simulink model "tadpole_dynamic_open_loop1"  (R2019b)
settings: Solver=ode4  StartTime=0.0  StopTime=sim_time  FixedStep=0.001  RelTol=1e-2
values from neighbouring files (symbols this model uses):
  C_alpha = 1000*ones(runcycle,1)    [rand_par.m]    (also in whole_par.m = 1000; whole_par_bias.m = 1000)
  C_beta = 50*ones(runcycle,1)    [rand_par.m]    (also in whole_par.m = 50; whole_par_bias.m = 50)
  Cd = 0.25*ones(runcycle,1)    [rand_par.m]    (also in whole_par.m = 0.25; whole_par_bias.m = 0.25)
  delta_fL = -1*ones(runcycle,1)    [rand_par.m]    (also in whole_par.m = -1; whole_par_bias.m = -1)
  delta_fR = 3.5*ones(runcycle,1)    [rand_par.m]    (also in whole_par.m = 3.5; whole_par_bias.m = 3.5)
  FA = 1*ones(runcycle,1)    [rand_par.m]    (also in whole_par.m = 1; whole_par_bias.m = 1)
  h = [ h(1:j-1) ; h(j+1:m)]    [UMDIRECT.m]    (also in whole_par.m = 0.4896; whole_par_bias.m = 0.4896)
  I_f_wheel = 0.3    [whole_par.m]    (also in whole_par_bias.m)
  I_r_wheel = 0.5    [whole_par.m]    (also in whole_par_bias.m)
  I_x = 12.1*ones(runcycle,1)    [rand_par.m]    (also in whole_par.m = 12.1; whole_par_bias.m = 12.1)
  I_y = 36.7*ones(runcycle,1)    [rand_par.m]    (also in whole_par.m = 36.7; whole_par_bias.m = 36.7)
  I_z = 50*DOE(:,2)    [rand_par.m]    (also in whole_par.m = 50; whole_par_bias.m = 60)
  k_z = 30000*ones(runcycle,1)    [rand_par.m]    (also in whole_par.m = 30000; whole_par_bias.m = 30000)
  l_1 = 0.724    [whole_par.m]    (also in whole_par_bias.m)
  l_2 = 0.719    [whole_par.m]    (also in whole_par_bias.m)
  m = m - 1    [UMDIRECT.m]    (also in rand_par.m = 48.3*DOE(:,1); whole_par.m = 48.3; whole_par_bias.m = 60)
  mu_dp = 0.8*ones(runcycle,1)    [rand_par.m]    (also in whole_par.m = 0.8; whole_par_bias.m = 0.8)
  mu_lp = 0.8*ones(runcycle,1)    [rand_par.m]    (also in whole_par.m = 0.8; whole_par_bias.m = 0.8)
  mu_rolling_1 = 0.009*ones(runcycle,1)    [rand_par.m]    (also in whole_par.m = 0.009; whole_par_bias.m = 0.009)
  mu_rolling_2 = 0.0005*ones(runcycle,1)    [rand_par.m]    (also in whole_par.m = 0.0005; whole_par_bias.m = 0.0005)
  R_0 = 0.335*ones(runcycle,1)    [rand_par.m]    (also in whole_par.m = 0.335; whole_par_bias.m = 0.335)
  rho = 1.225*ones(runcycle,1)    [rand_par.m]    (also in whole_par.m = 1.225; whole_par_bias.m = 1.225)
  SAP = 0.01*ones(runcycle,1)    [rand_par.m]    (also in whole_par.m = 0.01; whole_par_bias.m = 0.01)
  V_wind = 0*ones(runcycle,1)    [rand_par.m]    (also in whole_par.m = 0; whole_par_bias.m = 0)
libraries: simulink_extras x10, simulink x4
(part 3 of 4)

== system tadpole_dynamic_open_loop1/Vehicle Model/resistance calculation/Rear Traction add up/Fm<0/Switch Case Action Subsystem15 ==
  "value " : Inport
  Action Port : ActionPort  ActionPortLabel=case [ 1 ]:
  Merge1 : Merge  Inputs=3
  Switch Case Action Subsystem6 : Subsystem  TreatAsAtomicUnit=on
  Switch Case Action Subsystem7 : Subsystem  TreatAsAtomicUnit=on
  Switch Case Action Subsystem8 : Subsystem  TreatAsAtomicUnit=on
  Switch Case3 : SwitchCase  CaseConditions={1,-1}
  Out1 : Outport  VectorParamsAs1DForOutWhenUnconnected=off
  wires:
  Switch Case Action Subsystem7/1(Out1) -> Merge1/2
  Switch Case Action Subsystem6/1(Out1) -> Merge1/1
  [minus] -> Switch Case Action Subsystem7/1("value ")
  Switch Case Action Subsystem8/1(Out1) -> Merge1/3
  Switch Case3/2 -> Switch Case Action Subsystem7/Action  "m<b"
  [add] -> Switch Case Action Subsystem6/1("value ")
  Switch Case3/3 -> Switch Case Action Subsystem8/Action  "m=b"
  [minus] -> Switch Case Action Subsystem8/1("value ")
  Switch Case3/1 -> Switch Case Action Subsystem6/Action  "m>b"
  Merge1/1 -> Out1/1
  "value "/1 -> Switch Case3/1

== system tadpole_dynamic_open_loop1/Vehicle Model/resistance calculation/Rear Traction add up/Fm<0/Switch Case Action Subsystem6 ==
  "value " : Inport
  Action Port : ActionPort  ActionPortLabel=case [ -1 ]:
  Constant1 : Constant  Value=0
  Merge2 : Merge  Inputs=3
  Switch Case Action Subsystem10 : Subsystem  TreatAsAtomicUnit=on
  Switch Case Action Subsystem11 : Subsystem  TreatAsAtomicUnit=on
  Switch Case Action Subsystem9 : Subsystem  TreatAsAtomicUnit=on
  Switch Case4 : SwitchCase  CaseConditions={1,-1}
  Out1 : Outport  VectorParamsAs1DForOutWhenUnconnected=off
  wires:
  "value "/1 -> Switch Case4/1
  Switch Case4/2 -> Switch Case Action Subsystem10/Action  "m<b"
  [minus] -> Switch Case Action Subsystem10/1("value ")
  Switch Case Action Subsystem10/1(Out1) -> Merge2/2
  [add] -> Switch Case Action Subsystem9/1("value ")
  Switch Case4/1 -> Switch Case Action Subsystem9/Action  "m>b"
  Switch Case Action Subsystem9/1(Out1) -> Merge2/1
  Switch Case4/3 -> Switch Case Action Subsystem11/Action  "m=b"
  Constant1/1 -> Switch Case Action Subsystem11/1("value ")
  Switch Case Action Subsystem11/1(Out1) -> Merge2/3
  Merge2/1 -> Out1/1

== system tadpole_dynamic_open_loop1/Vehicle Model/resistance calculation/Rear Traction add up/Fm<0/Switch Case Action Subsystem7 ==
  "value " : Inport
  Action Port : ActionPort  ActionPortLabel=default:
  Constant1 : Constant  Value=0
  Constant2 : Constant  Value=0
  Merge3 : Merge  Inputs=3
  Switch Case Action Subsystem12 : Subsystem  TreatAsAtomicUnit=on
  Switch Case Action Subsystem13 : Subsystem  TreatAsAtomicUnit=on
  Switch Case Action Subsystem14 : Subsystem  TreatAsAtomicUnit=on
  Switch Case5 : SwitchCase  CaseConditions={1,-1}
  Out1 : Outport  VectorParamsAs1DForOutWhenUnconnected=off
  wires:
  "value "/1 -> Switch Case5/1
  Switch Case5/1 -> Switch Case Action Subsystem14/Action  "m>b"
  Switch Case Action Subsystem14/1(Out1) -> Merge3/1
  Switch Case Action Subsystem12/1(Out1) -> Merge3/2
  Constant1/1 -> Switch Case Action Subsystem12/1("value ")
  Switch Case Action Subsystem13/1(Out1) -> Merge3/3
  Switch Case5/3 -> Switch Case Action Subsystem13/Action  "m=b"
  Switch Case5/2 -> Switch Case Action Subsystem12/Action  "m<b"
  [add] -> Switch Case Action Subsystem14/1("value ")
  Constant2/1 -> Switch Case Action Subsystem13/1("value ")
  Merge3/1 -> Out1/1

== system tadpole_dynamic_open_loop1/Vehicle Model/resistance calculation/Rear Traction add up/Fm>=0/Switch Case Action Subsystem6 ==
  "value " : Inport
  In2 : Inport  Port=2
  In3 : Inport  Port=3
  Action Port : ActionPort  ActionPortLabel=case [ -1 ]:
  Constant : Constant  Value=2
  Constant1 : Constant  Value=0
  Merge2 : Merge  Inputs=3
  Switch Case Action Subsystem10 : Subsystem  TreatAsAtomicUnit=on
  Switch Case Action Subsystem11 : Subsystem  TreatAsAtomicUnit=on
  Switch Case Action Subsystem9 : Subsystem  TreatAsAtomicUnit=on
  Switch Case4 : SwitchCase  CaseConditions={1,-1}
  Out1 : Outport  VectorParamsAs1DForOutWhenUnconnected=off
  Out2 : Outport  Port=2  VectorParamsAs1DForOutWhenUnconnected=off
  wires:
  "value "/1 -> Switch Case4/1
  Switch Case4/2 -> Switch Case Action Subsystem10/Action  "V-"
  [minus_2] -> Switch Case Action Subsystem10/1("value ")
  Switch Case Action Subsystem10/1(Out1) -> Merge2/2
  [minus_2] -> Switch Case Action Subsystem9/1("value ")
  Switch Case4/1 -> Switch Case Action Subsystem9/Action  "V+"
  Switch Case Action Subsystem9/1(Out1) -> Merge2/1
  Switch Case4/3 -> Switch Case Action Subsystem11/Action  "V=0"
  Constant1/1 -> Switch Case Action Subsystem11/1("value ")
  Switch Case Action Subsystem11/1(Out1) -> Merge2/3
  Merge2/1 -> Out1/1
  In2/1 -> [add_2]
  In3/1 -> [minus_2]
  Constant/1 -> Out2/1

== system tadpole_dynamic_open_loop1/Vehicle Model/resistance calculation/Rear Traction add up/Fm>=0/Switch Case Action Subsystem7 ==
  "value " : Inport
  In2 : Inport  Port=2
  In3 : Inport  Port=3
  Action Port : ActionPort  ActionPortLabel=default:
  Constant : Constant  Value=3
  Constant2 : Constant  Value=0
  Merge3 : Merge  Inputs=3
  Switch Case Action Subsystem12 : Subsystem  TreatAsAtomicUnit=on
  Switch Case Action Subsystem13 : Subsystem  TreatAsAtomicUnit=on
  Switch Case Action Subsystem14 : Subsystem  TreatAsAtomicUnit=on
  Switch Case5 : SwitchCase  CaseConditions={1,-1}
  Out1 : Outport  VectorParamsAs1DForOutWhenUnconnected=off
  Out2 : Outport  Port=2  VectorParamsAs1DForOutWhenUnconnected=off
  wires:
  "value "/1 -> Switch Case5/1
  Switch Case5/1 -> Switch Case Action Subsystem14/Action  "m>b"
  Switch Case Action Subsystem14/1(Out1) -> Merge3/1
  Switch Case Action Subsystem12/1(Out1) -> Merge3/2
  [minus_3] -> Switch Case Action Subsystem12/1("value ")
  Switch Case Action Subsystem13/1(Out1) -> Merge3/3
  Switch Case5/3 -> Switch Case Action Subsystem13/Action  "m=b"
  Switch Case5/2 -> Switch Case Action Subsystem12/Action  "m<b"
  [minus_3] -> Switch Case Action Subsystem14/1("value ")
  Constant2/1 -> Switch Case Action Subsystem13/1("value ")
  Merge3/1 -> Out1/1
  In2/1 -> [add_3]
  In3/1 -> [minus_3]
  Constant/1 -> Out2/1

== system tadpole_dynamic_open_loop1/Vehicle Model/resistance calculation/Rear Traction add up/Fm>=0/m>b ==
  "velocity sign " : Inport
  add : Inport  Port=2
  "minus " : Inport  Port=3
  Action Port : ActionPort  ActionPortLabel=case [ 1 ]:
  Constant : Constant
  Merge1 : Merge  Inputs=3
  Switch Case Action Subsystem6 : Subsystem  TreatAsAtomicUnit=on
  Switch Case Action Subsystem7 : Subsystem  TreatAsAtomicUnit=on
  Switch Case Action Subsystem8 : Subsystem  TreatAsAtomicUnit=on
  Switch Case3 : SwitchCase  CaseConditions={1,-1}
  Out1 : Outport  VectorParamsAs1DForOutWhenUnconnected=off
  Out2 : Outport  Port=2  VectorParamsAs1DForOutWhenUnconnected=off
  wires:
  Switch Case Action Subsystem7/1(Out1) -> Merge1/2
  Switch Case Action Subsystem6/1(Out1) -> Merge1/1
  [add_1] -> Switch Case Action Subsystem7/1("value ")
  Switch Case Action Subsystem8/1(Out1) -> Merge1/3
  Switch Case3/2 -> Switch Case Action Subsystem7/Action  "V-"
  [minus_1] -> Switch Case Action Subsystem6/1("value ")
  Switch Case3/3 -> Switch Case Action Subsystem8/Action  "V=0"
  [minus_1] -> Switch Case Action Subsystem8/1("value ")
  Switch Case3/1 -> Switch Case Action Subsystem6/Action  "V+"
  Merge1/1 -> Out1/1
  "velocity sign "/1 -> Switch Case3/1
  add/1 -> [add_1]
  "minus "/1 -> [minus_1]
  Constant/1 -> Out2/1

== system tadpole_dynamic_open_loop1/Vehicle Model/resistance calculation/Rolling Resistance Force Front L/Subsystem/w_1 ==
  In : Inport
  Product : Product
  Out : Outport  VectorParamsAs1DForOutWhenUnconnected=off
  wires:
  [w_1] -> Product/2
  Product/1 -> Out/1
  In/1 -> Product/1

== system tadpole_dynamic_open_loop1/Vehicle Model/resistance calculation/Rolling Resistance Force Front R/Subsystem/w_2 ==
  In : Inport
  Product : Product
  Out : Outport  VectorParamsAs1DForOutWhenUnconnected=off
  wires:
  [w_2] -> Product/2
  Product/1 -> Out/1
  In/1 -> Product/1

== system tadpole_dynamic_open_loop1/Vehicle Model/resistance calculation/linear slip cal. /slip recgonition/If Action Subsystem ==
  In1 : Inport
  Action Port : ActionPort  ActionPortLabel=if(u1~=0)
  Out1 : Outport  VectorParamsAs1DForOutWhenUnconnected=off
  wires:
  In1/1 -> Out1/1

== system tadpole_dynamic_open_loop1/Vehicle Model/resistance calculation/linear slip cal. /slip recgonition/If Action Subsystem1 ==
  In1 : Inport
  Action Port : ActionPort  ActionPortLabel=else
  Out1 : Outport  VectorParamsAs1DForOutWhenUnconnected=off
  wires:
  In1/1 -> Out1/1

== system tadpole_dynamic_open_loop1/Vehicle Model/resistance calculation/velocity limit x/If Action Subsystem2/If Action Subsystem ==
  In1 : Inport
  Action Port : ActionPort  ActionPortLabel=if(0.005>u1 )
  Out1 : Outport  VectorParamsAs1DForOutWhenUnconnected=off
  wires:
  In1/1 -> Out1/1

== system tadpole_dynamic_open_loop1/Vehicle Model/resistance calculation/velocity limit x/If Action Subsystem2/If Action Subsystem1 ==
  In1 : Inport
  Action Port : ActionPort  ActionPortLabel=else
  Out1 : Outport  VectorParamsAs1DForOutWhenUnconnected=off
  wires:
  In1/1 -> Out1/1

== system tadpole_dynamic_open_loop1/Vehicle Model/resistance calculation/velocity limit x/If Action Subsystem3/If Action Subsystem ==
  In1 : Inport
  Action Port : ActionPort  ActionPortLabel=if(-0.005<u1 )
  Out1 : Outport  VectorParamsAs1DForOutWhenUnconnected=off
  wires:
  In1/1 -> Out1/1

== system tadpole_dynamic_open_loop1/Vehicle Model/resistance calculation/velocity limit x/If Action Subsystem3/If Action Subsystem1 ==
  In1 : Inport
  Action Port : ActionPort  ActionPortLabel=else
  Out1 : Outport  VectorParamsAs1DForOutWhenUnconnected=off
  wires:
  In1/1 -> Out1/1

== system tadpole_dynamic_open_loop1/Vehicle Model/resistance calculation/velocity limit y/If Action Subsystem2/If Action Subsystem ==
  In1 : Inport
  Action Port : ActionPort  ActionPortLabel=if(0.005>u1 )
  Out1 : Outport  VectorParamsAs1DForOutWhenUnconnected=off
  wires:
  In1/1 -> Out1/1

== system tadpole_dynamic_open_loop1/Vehicle Model/resistance calculation/velocity limit y/If Action Subsystem2/If Action Subsystem1 ==
  In1 : Inport
  Action Port : ActionPort  ActionPortLabel=else
  Out1 : Outport  VectorParamsAs1DForOutWhenUnconnected=off
  wires:
  In1/1 -> Out1/1

== system tadpole_dynamic_open_loop1/Vehicle Model/resistance calculation/velocity limit y/If Action Subsystem3/If Action Subsystem ==
  In1 : Inport
  Action Port : ActionPort  ActionPortLabel=if(-0.005<u1 )
  Out1 : Outport  VectorParamsAs1DForOutWhenUnconnected=off
  wires:
  In1/1 -> Out1/1

== system tadpole_dynamic_open_loop1/Vehicle Model/resistance calculation/velocity limit y/If Action Subsystem3/If Action Subsystem1 ==
  In1 : Inport
  Action Port : ActionPort  ActionPortLabel=else
  Out1 : Outport  VectorParamsAs1DForOutWhenUnconnected=off
  wires:
  In1/1 -> Out1/1

== system tadpole_dynamic_open_loop1/Vehicle Model/Tadpole vehicle dynamic/Calculation/Side slip angle Rear/velocity limit1/If Action Subsystem2 ==
  In1 : Inport
  Action Port : ActionPort  ActionPortLabel=if(u1>0 )
  Constant : Constant  Value=0
  If : If  IfExpression=0.0005>u1
  If Action Subsystem : Subsystem  TreatAsAtomicUnit=on
  If Action Subsystem1 : Subsystem  TreatAsAtomicUnit=on
  Merge : Merge
  Out1 : Outport  VectorParamsAs1DForOutWhenUnconnected=off
  wires:
  Merge/1 -> Out1/1
  If Action Subsystem1/1(Out1) -> Merge/2
  If Action Subsystem/1(Out1) -> Merge/1
  Constant/1 -> If Action Subsystem/1(In1)
  If/2 -> If Action Subsystem1/Action
  If/1 -> If Action Subsystem/Action
  In1/1 -> If Action Subsystem1/1(In1), If/1

== system tadpole_dynamic_open_loop1/Vehicle Model/Tadpole vehicle dynamic/Calculation/Side slip angle Rear/velocity limit1/If Action Subsystem3 ==
  In1 : Inport
  Action Port : ActionPort  ActionPortLabel=else
  Constant : Constant  Value=0
  If : If  IfExpression=-0.0005<u1
  If Action Subsystem : Subsystem  TreatAsAtomicUnit=on
  If Action Subsystem1 : Subsystem  TreatAsAtomicUnit=on
  Merge : Merge
  Out1 : Outport  VectorParamsAs1DForOutWhenUnconnected=off
  wires:
  In1/1 -> If/1, If Action Subsystem1/1(In1)
  If/1 -> If Action Subsystem/Action
  If/2 -> If Action Subsystem1/Action
  Constant/1 -> If Action Subsystem/1(In1)
  If Action Subsystem/1(Out1) -> Merge/1
  If Action Subsystem1/1(Out1) -> Merge/2
  Merge/1 -> Out1/1

== system tadpole_dynamic_open_loop1/Vehicle Model/Tadpole vehicle dynamic/Calculation/Subsystem1/Subsystem/linear slip cal fR  ==
  Lateral Force : Inport
  Normal Force : Inport  Port=2
  MinMax : MinMax  Inputs=2
  Product : Product
  Subtract : Sum  Inputs=+-
  Switch : Switch  Criteria=u2 > Threshold
  max. lat. friction coefficient : Constant  Value=mu_lp
  slip recgonition : Subsystem
  Lateral force : Outport  VectorParamsAs1DForOutWhenUnconnected=off
  wires:
  Subtract/1 -> Switch/2
  Product/1 -> Switch/3, Subtract/2, slip recgonition/1(In2), MinMax/1
  max. lat. friction coefficient/1 -> Product/1
  MinMax/1 -> slip recgonition/2(In3)
  Lateral Force/1 -> Switch/1, Subtract/1, MinMax/2
  Normal Force/1 -> Product/2
  Switch/1 -> Lateral force/1

== system tadpole_dynamic_open_loop1/Vehicle Model/Tadpole vehicle dynamic/Calculation/Subsystem1/velocity limit/If Action Subsystem2 ==
  In1 : Inport
  Action Port : ActionPort
  Constant : Constant  Value=0
  If : If  IfExpression=0.005>u1
  If Action Subsystem : Subsystem  TreatAsAtomicUnit=on
  If Action Subsystem1 : Subsystem  TreatAsAtomicUnit=on
  Merge : Merge
  Out1 : Outport  VectorParamsAs1DForOutWhenUnconnected=off
  wires:
  Merge/1 -> Out1/1
  If Action Subsystem1/1(Out1) -> Merge/2
  If Action Subsystem/1(Out1) -> Merge/1
  Constant/1 -> If Action Subsystem/1(In1)
  If/2 -> If Action Subsystem1/Action
  If/1 -> If Action Subsystem/Action
  In1/1 -> If Action Subsystem1/1(In1), If/1

== system tadpole_dynamic_open_loop1/Vehicle Model/Tadpole vehicle dynamic/Calculation/Subsystem1/velocity limit/If Action Subsystem3 ==
  In1 : Inport
  Action Port : ActionPort
  Constant : Constant  Value=0
  If : If  IfExpression=-0.005<u1
  If Action Subsystem : Subsystem  TreatAsAtomicUnit=on
  If Action Subsystem1 : Subsystem  TreatAsAtomicUnit=on
  Merge : Merge
  Out1 : Outport  VectorParamsAs1DForOutWhenUnconnected=off
  wires:
  In1/1 -> If Action Subsystem1/1(In1), If/1
  If/1 -> If Action Subsystem/Action
  If/2 -> If Action Subsystem1/Action
  Constant/1 -> If Action Subsystem/1(In1)
  If Action Subsystem/1(Out1) -> Merge/1
  If Action Subsystem1/1(Out1) -> Merge/2
  Merge/1 -> Out1/1

== system tadpole_dynamic_open_loop1/Vehicle Model/Tadpole vehicle dynamic/Calculation/Subsystem2/Subsystem/linear slip cal r  ==
  Lateral Force : Inport
  Normal Force : Inport  Port=2
  MinMax : MinMax  Inputs=2
  Product : Product
  Subtract : Sum  Inputs=+-
  Switch : Switch  Criteria=u2 > Threshold
  max. lat. friction coefficient : Constant  Value=mu_lp
  slip recgonition : Subsystem
  Lateral force : Outport  VectorParamsAs1DForOutWhenUnconnected=off
  wires:
  Product/1 -> Switch/3, Subtract/2, slip recgonition/1(In2), MinMax/1
  MinMax/1 -> slip recgonition/2(In3)
  Switch/1 -> Lateral force/1
  Lateral Force/1 -> Switch/1, Subtract/1, MinMax/2
  Normal Force/1 -> Product/2
  max. lat. friction coefficient/1 -> Product/1
  Subtract/1 -> Switch/2

== system tadpole_dynamic_open_loop1/Vehicle Model/Tadpole vehicle dynamic/Calculation/Subsystem2/velocity limit/If Action Subsystem2 ==
  In1 : Inport
  Action Port : ActionPort
  Constant : Constant  Value=0
  If : If  IfExpression=0.005>u1
  If Action Subsystem : Subsystem  TreatAsAtomicUnit=on
  If Action Subsystem1 : Subsystem  TreatAsAtomicUnit=on
  Merge : Merge
  Out1 : Outport  VectorParamsAs1DForOutWhenUnconnected=off
  wires:
  Merge/1 -> Out1/1
  If Action Subsystem1/1(Out1) -> Merge/2
  If Action Subsystem/1(Out1) -> Merge/1
  Constant/1 -> If Action Subsystem/1(In1)
  If/2 -> If Action Subsystem1/Action
  If/1 -> If Action Subsystem/Action
  In1/1 -> If Action Subsystem1/1(In1), If/1

== system tadpole_dynamic_open_loop1/Vehicle Model/Tadpole vehicle dynamic/Calculation/Subsystem2/velocity limit/If Action Subsystem3 ==
  In1 : Inport
  Action Port : ActionPort
  Constant : Constant  Value=0
  If : If  IfExpression=-0.005<u1
  If Action Subsystem : Subsystem  TreatAsAtomicUnit=on
  If Action Subsystem1 : Subsystem  TreatAsAtomicUnit=on
  Merge : Merge
  Out1 : Outport  VectorParamsAs1DForOutWhenUnconnected=off
  wires:
  In1/1 -> If Action Subsystem1/1(In1), If/1
  If/1 -> If Action Subsystem/Action
  If/2 -> If Action Subsystem1/Action
  Constant/1 -> If Action Subsystem/1(In1)
  If Action Subsystem/1(Out1) -> Merge/1
  If Action Subsystem1/1(Out1) -> Merge/2
  Merge/1 -> Out1/1

== system tadpole_dynamic_open_loop1/Vehicle Model/Tadpole vehicle dynamic/Calculation/Subsystem3/Subsystem/linear slip cal fL  ==
  Lateral Force : Inport
  Normal Force : Inport  Port=2
  MinMax : MinMax  Inputs=2
  Product : Product
  Subtract : Sum  Inputs=+-
  Switch : Switch  Criteria=u2 > Threshold
  max. lat. friction coefficient : Constant  Value=mu_lp
  slip recgonition : Subsystem
  Lateral force : Outport  VectorParamsAs1DForOutWhenUnconnected=off
  wires:
  Subtract/1 -> Switch/2
  Product/1 -> Switch/3, Subtract/2, slip recgonition/1(In2), MinMax/1
  max. lat. friction coefficient/1 -> Product/1
  MinMax/1 -> slip recgonition/2(In3)
  Lateral Force/1 -> Switch/1, Subtract/1, MinMax/2
  Normal Force/1 -> Product/2
  Switch/1 -> Lateral force/1

== system tadpole_dynamic_open_loop1/Vehicle Model/Tadpole vehicle dynamic/Calculation/Subsystem3/velocity limit/If Action Subsystem2 ==
  In1 : Inport
  Action Port : ActionPort
  Constant : Constant  Value=0
  If : If  IfExpression=0.005>u1
  If Action Subsystem : Subsystem  TreatAsAtomicUnit=on
  If Action Subsystem1 : Subsystem  TreatAsAtomicUnit=on
  Merge : Merge
  Out1 : Outport  VectorParamsAs1DForOutWhenUnconnected=off
  wires:
  Merge/1 -> Out1/1
  If Action Subsystem1/1(Out1) -> Merge/2
  If Action Subsystem/1(Out1) -> Merge/1
  Constant/1 -> If Action Subsystem/1(In1)
  If/2 -> If Action Subsystem1/Action
  If/1 -> If Action Subsystem/Action
  In1/1 -> If Action Subsystem1/1(In1), If/1

== system tadpole_dynamic_open_loop1/Vehicle Model/Tadpole vehicle dynamic/Calculation/Subsystem3/velocity limit/If Action Subsystem3 ==
  In1 : Inport
  Action Port : ActionPort
  Constant : Constant  Value=0
  If : If  IfExpression=-0.005<u1
  If Action Subsystem : Subsystem  TreatAsAtomicUnit=on
  If Action Subsystem1 : Subsystem  TreatAsAtomicUnit=on
  Merge : Merge
  Out1 : Outport  VectorParamsAs1DForOutWhenUnconnected=off
  wires:
  In1/1 -> If Action Subsystem1/1(In1), If/1
  If/1 -> If Action Subsystem/Action
  If/2 -> If Action Subsystem1/Action
  Constant/1 -> If Action Subsystem/1(In1)
  If Action Subsystem/1(Out1) -> Merge/1
  If Action Subsystem1/1(Out1) -> Merge/2
  Merge/1 -> Out1/1

== system tadpole_dynamic_open_loop1/Vehicle Model/Tadpole vehicle dynamic/Calculation/Subsystem4/Subsystem/linear slip cal fR  ==
  Lateral Force : Inport
  Normal Force : Inport  Port=2
  Gain2 : Gain  Gain=-1
  MinMax : MinMax  Inputs=2
  MinMax2 : MinMax  Function=max  Inputs=2
  Product : Product
  max. lat. friction coefficient : Constant  Value=mu_lp
  slip recgonition : Subsystem
  Lateral force : Outport  VectorParamsAs1DForOutWhenUnconnected=off
  wires:
  Gain2/1 -> MinMax2/2
  Product/1 -> Gain2/1, slip recgonition/1(In2), MinMax/1
  MinMax/1 -> slip recgonition/2(In3), MinMax2/1
  MinMax2/1 -> Lateral force/1
  Lateral Force/1 -> MinMax/2
  Normal Force/1 -> Product/2
  max. lat. friction coefficient/1 -> Product/1

== system tadpole_dynamic_open_loop1/Vehicle Model/Tadpole vehicle dynamic/Calculation/Subsystem4/velocity limit/If Action Subsystem2 ==
  In1 : Inport
  Action Port : ActionPort  ActionPortLabel=if(u1>0 )
  Constant : Constant  Value=0
  If : If  IfExpression=0.005>u1
  If Action Subsystem : Subsystem  TreatAsAtomicUnit=on
  If Action Subsystem1 : Subsystem  TreatAsAtomicUnit=on
  Merge : Merge
  Out1 : Outport  VectorParamsAs1DForOutWhenUnconnected=off
  wires:
  Merge/1 -> Out1/1
  If Action Subsystem1/1(Out1) -> Merge/2
  If Action Subsystem/1(Out1) -> Merge/1
  Constant/1 -> If Action Subsystem/1(In1)
  If/2 -> If Action Subsystem1/Action
  If/1 -> If Action Subsystem/Action
  In1/1 -> If Action Subsystem1/1(In1), If/1

== system tadpole_dynamic_open_loop1/Vehicle Model/Tadpole vehicle dynamic/Calculation/Subsystem4/velocity limit/If Action Subsystem3 ==
  In1 : Inport
  Action Port : ActionPort  ActionPortLabel=else
  Constant : Constant  Value=0
  If : If  IfExpression=-0.005<u1
  If Action Subsystem : Subsystem  TreatAsAtomicUnit=on
  If Action Subsystem1 : Subsystem  TreatAsAtomicUnit=on
  Merge : Merge
  Out1 : Outport  VectorParamsAs1DForOutWhenUnconnected=off
  wires:
  In1/1 -> If Action Subsystem1/1(In1), If/1
  If/1 -> If Action Subsystem/Action
  If/2 -> If Action Subsystem1/Action
  Constant/1 -> If Action Subsystem/1(In1)
  If Action Subsystem/1(Out1) -> Merge/1
  If Action Subsystem1/1(Out1) -> Merge/2
  Merge/1 -> Out1/1

== system tadpole_dynamic_open_loop1/Vehicle Model/Tadpole vehicle dynamic/Calculation/Subsystem5/Subsystem/linear slip cal r  ==
  Lateral Force : Inport
  Normal Force : Inport  Port=2
  MinMax : MinMax  Inputs=2
  MinMax2 : MinMax  Function=max  Inputs=2
  Product : Product
  max. lat. friction coefficient : Constant  Value=mu_lp
  multiply -1 : MATLAB Function  TreatAsAtomicUnit=on
  slip recgonition : Subsystem
  Lateral force : Outport  VectorParamsAs1DForOutWhenUnconnected=off
  wires:
  multiply -1/1(y) -> MinMax2/2
  MinMax/1 -> slip recgonition/2(In3), MinMax2/1
  Lateral Force/1 -> MinMax/2
  Normal Force/1 -> Product/2
  max. lat. friction coefficient/1 -> Product/1
  MinMax2/1 -> Lateral force/1
  Product/1 -> multiply -1/1(u), slip recgonition/1(In2), MinMax/1

== system tadpole_dynamic_open_loop1/Vehicle Model/Tadpole vehicle dynamic/Calculation/Subsystem5/velocity limit/If Action Subsystem2 ==
  In1 : Inport
  Action Port : ActionPort  ActionPortLabel=if(u1>0 )
  Constant : Constant  Value=0
  If : If  IfExpression=0.005>u1
  If Action Subsystem : Subsystem  TreatAsAtomicUnit=on
  If Action Subsystem1 : Subsystem  TreatAsAtomicUnit=on
  Merge : Merge
  Out1 : Outport  VectorParamsAs1DForOutWhenUnconnected=off
  wires:
  Merge/1 -> Out1/1
  If Action Subsystem1/1(Out1) -> Merge/2
  If Action Subsystem/1(Out1) -> Merge/1
  Constant/1 -> If Action Subsystem/1(In1)
  If/2 -> If Action Subsystem1/Action
  If/1 -> If Action Subsystem/Action
  In1/1 -> If Action Subsystem1/1(In1), If/1

== system tadpole_dynamic_open_loop1/Vehicle Model/Tadpole vehicle dynamic/Calculation/Subsystem5/velocity limit/If Action Subsystem3 ==
  In1 : Inport
  Action Port : ActionPort  ActionPortLabel=else
  Constant : Constant  Value=0
  If : If  IfExpression=-0.005<u1
  If Action Subsystem : Subsystem  TreatAsAtomicUnit=on
  If Action Subsystem1 : Subsystem  TreatAsAtomicUnit=on
  Merge : Merge
  Out1 : Outport  VectorParamsAs1DForOutWhenUnconnected=off
  wires:
  In1/1 -> If Action Subsystem1/1(In1), If/1
  If/1 -> If Action Subsystem/Action
  If/2 -> If Action Subsystem1/Action
  Constant/1 -> If Action Subsystem/1(In1)
  If Action Subsystem/1(Out1) -> Merge/1
  If Action Subsystem1/1(Out1) -> Merge/2
  Merge/1 -> Out1/1

== system tadpole_dynamic_open_loop1/Vehicle Model/Tadpole vehicle dynamic/Calculation/Subsystem6/Subsystem/linear slip cal fL  ==
  Lateral Force : Inport
  Normal Force : Inport  Port=2
  Gain2 : Gain  Gain=-1
  MinMax : MinMax  Inputs=2
  MinMax2 : MinMax  Function=max  Inputs=2
  Product : Product
  max. lat. friction coefficient : Constant  Value=mu_lp
  slip recgonition : Subsystem
  Lateral force : Outport  VectorParamsAs1DForOutWhenUnconnected=off
  wires:
  Gain2/1 -> MinMax2/2
  Product/1 -> Gain2/1, slip recgonition/1(In2), MinMax/1
  MinMax/1 -> slip recgonition/2(In3), MinMax2/1
  MinMax2/1 -> Lateral force/1
  Lateral Force/1 -> MinMax/2
  Normal Force/1 -> Product/2
  max. lat. friction coefficient/1 -> Product/1

== system tadpole_dynamic_open_loop1/Vehicle Model/Tadpole vehicle dynamic/Calculation/Subsystem6/velocity limit/If Action Subsystem2 ==
  In1 : Inport
  Action Port : ActionPort  ActionPortLabel=if(u1>0 )
  Constant : Constant  Value=0
  If : If  IfExpression=0.005>u1
  If Action Subsystem : Subsystem  TreatAsAtomicUnit=on
  If Action Subsystem1 : Subsystem  TreatAsAtomicUnit=on
  Merge : Merge
  Out1 : Outport  VectorParamsAs1DForOutWhenUnconnected=off
  wires:
  Merge/1 -> Out1/1
  If Action Subsystem1/1(Out1) -> Merge/2
  If Action Subsystem/1(Out1) -> Merge/1
  Constant/1 -> If Action Subsystem/1(In1)
  If/2 -> If Action Subsystem1/Action
  If/1 -> If Action Subsystem/Action
  In1/1 -> If Action Subsystem1/1(In1), If/1

== system tadpole_dynamic_open_loop1/Vehicle Model/Tadpole vehicle dynamic/Calculation/Subsystem6/velocity limit/If Action Subsystem3 ==
  In1 : Inport
  Action Port : ActionPort  ActionPortLabel=else
  Constant : Constant  Value=0
  If : If  IfExpression=-0.005<u1
  If Action Subsystem : Subsystem  TreatAsAtomicUnit=on
  If Action Subsystem1 : Subsystem  TreatAsAtomicUnit=on
  Merge : Merge
  Out1 : Outport  VectorParamsAs1DForOutWhenUnconnected=off
  wires:
  In1/1 -> If Action Subsystem1/1(In1), If/1
  If/1 -> If Action Subsystem/Action
  If/2 -> If Action Subsystem1/Action
  Constant/1 -> If Action Subsystem/1(In1)
  If Action Subsystem/1(Out1) -> Merge/1
  If Action Subsystem1/1(Out1) -> Merge/2
  Merge/1 -> Out1/1

== system tadpole_dynamic_open_loop1/Vehicle Model/Tadpole vehicle dynamic/Calculation/side slip angle Front/velocity limit1/If Action Subsystem2 ==
  In1 : Inport
  Action Port : ActionPort  ActionPortLabel=if(u1>0 )
  Constant : Constant  Value=0
  If : If  IfExpression=0.0005>u1
  If Action Subsystem : Subsystem  TreatAsAtomicUnit=on
  If Action Subsystem1 : Subsystem  TreatAsAtomicUnit=on
  Merge : Merge
  Out1 : Outport  VectorParamsAs1DForOutWhenUnconnected=off
  wires:
  Merge/1 -> Out1/1
  If Action Subsystem1/1(Out1) -> Merge/2
  If Action Subsystem/1(Out1) -> Merge/1
  Constant/1 -> If Action Subsystem/1(In1)
  If/2 -> If Action Subsystem1/Action
  If/1 -> If Action Subsystem/Action
  In1/1 -> If Action Subsystem1/1(In1), If/1

== system tadpole_dynamic_open_loop1/Vehicle Model/Tadpole vehicle dynamic/Calculation/side slip angle Front/velocity limit1/If Action Subsystem3 ==
  In1 : Inport
  Action Port : ActionPort  ActionPortLabel=else
  Constant : Constant  Value=0
  If : If  IfExpression=-0.0005<u1
  If Action Subsystem : Subsystem  TreatAsAtomicUnit=on
  If Action Subsystem1 : Subsystem  TreatAsAtomicUnit=on
  Merge : Merge
  Out1 : Outport  VectorParamsAs1DForOutWhenUnconnected=off
  wires:
  In1/1 -> If/1, If Action Subsystem1/1(In1)
  If/1 -> If Action Subsystem/Action
  If/2 -> If Action Subsystem1/Action
  Constant/1 -> If Action Subsystem/1(In1)
  If Action Subsystem/1(Out1) -> Merge/1
  If Action Subsystem1/1(Out1) -> Merge/2
  Merge/1 -> Out1/1

== system tadpole_dynamic_open_loop1/Vehicle Model/Tadpole vehicle dynamic/Calculation/side slip angle Front/velocity limit2/If Action Subsystem2 ==
  In1 : Inport
  Action Port : ActionPort  ActionPortLabel=if(u1>0 )
  Constant : Constant  Value=0
  If : If  IfExpression=0.0005>u1
  If Action Subsystem : Subsystem  TreatAsAtomicUnit=on
  If Action Subsystem1 : Subsystem  TreatAsAtomicUnit=on
  Merge : Merge
  Out1 : Outport  VectorParamsAs1DForOutWhenUnconnected=off
  wires:
  Merge/1 -> Out1/1
  If Action Subsystem1/1(Out1) -> Merge/2
  If Action Subsystem/1(Out1) -> Merge/1
  Constant/1 -> If Action Subsystem/1(In1)
  If/2 -> If Action Subsystem1/Action
  If/1 -> If Action Subsystem/Action
  In1/1 -> If Action Subsystem1/1(In1), If/1

== system tadpole_dynamic_open_loop1/Vehicle Model/Tadpole vehicle dynamic/Calculation/side slip angle Front/velocity limit2/If Action Subsystem3 ==
  In1 : Inport
  Action Port : ActionPort  ActionPortLabel=else
  Constant : Constant  Value=0
  If : If  IfExpression=-0.0005<u1
  If Action Subsystem : Subsystem  TreatAsAtomicUnit=on
  If Action Subsystem1 : Subsystem  TreatAsAtomicUnit=on
  Merge : Merge
  Out1 : Outport  VectorParamsAs1DForOutWhenUnconnected=off
  wires:
  In1/1 -> If/1, If Action Subsystem1/1(In1)
  If/1 -> If Action Subsystem/Action
  If/2 -> If Action Subsystem1/Action
  Constant/1 -> If Action Subsystem/1(In1)
  If Action Subsystem/1(Out1) -> Merge/1
  If Action Subsystem1/1(Out1) -> Merge/2
  Merge/1 -> Out1/1

== system tadpole_dynamic_open_loop1/Vehicle Model/Tadpole vehicle dynamic/Calculation/velocity limit1/If Action Subsystem2/If Action Subsystem ==
  In1 : Inport
  Action Port : ActionPort  ActionPortLabel=if(0.005>u1 )
  Out1 : Outport  VectorParamsAs1DForOutWhenUnconnected=off
  wires:
  In1/1 -> Out1/1

== system tadpole_dynamic_open_loop1/Vehicle Model/Tadpole vehicle dynamic/Calculation/velocity limit1/If Action Subsystem2/If Action Subsystem1 ==
  In1 : Inport
  Action Port : ActionPort  ActionPortLabel=else
  Out1 : Outport  VectorParamsAs1DForOutWhenUnconnected=off
  wires:
  In1/1 -> Out1/1

== system tadpole_dynamic_open_loop1/Vehicle Model/Tadpole vehicle dynamic/Calculation/velocity limit1/If Action Subsystem3/If Action Subsystem ==
  In1 : Inport
  Action Port : ActionPort  ActionPortLabel=if(-0.005<u1 )
  Out1 : Outport  VectorParamsAs1DForOutWhenUnconnected=off
  wires:
  In1/1 -> Out1/1

== system tadpole_dynamic_open_loop1/Vehicle Model/Tadpole vehicle dynamic/Calculation/velocity limit1/If Action Subsystem3/If Action Subsystem1 ==
  In1 : Inport
  Action Port : ActionPort  ActionPortLabel=else
  Out1 : Outport  VectorParamsAs1DForOutWhenUnconnected=off
  wires:
  In1/1 -> Out1/1

== system tadpole_dynamic_open_loop1/Vehicle Model/resistance calculation/Rear Traction add up/Fm<0/Switch Case Action Subsystem15/Switch Case Action Subsystem6 ==
  "value " : Inport
  Action Port : ActionPort  ActionPortLabel=case [ 1 ]:
  Gain : Gain  Gain=-1
  Out1 : Outport  VectorParamsAs1DForOutWhenUnconnected=off
  wires:
  "value "/1 -> Gain/1
  Gain/1 -> Out1/1

== system tadpole_dynamic_open_loop1/Vehicle Model/resistance calculation/Rear Traction add up/Fm<0/Switch Case Action Subsystem15/Switch Case Action Subsystem7 ==
  "value " : Inport
  Action Port : ActionPort  ActionPortLabel=case [ -1 ]:
  Gain : Gain  Gain=-1
  Out1 : Outport  VectorParamsAs1DForOutWhenUnconnected=off
  wires:
  "value "/1 -> Gain/1
  Gain/1 -> Out1/1

== system tadpole_dynamic_open_loop1/Vehicle Model/resistance calculation/Rear Traction add up/Fm<0/Switch Case Action Subsystem15/Switch Case Action Subsystem8 ==
  "value " : Inport
  Action Port : ActionPort  ActionPortLabel=default:
  Gain : Gain  Gain=-1
  Out1 : Outport  VectorParamsAs1DForOutWhenUnconnected=off
  wires:
  "value "/1 -> Gain/1
  Gain/1 -> Out1/1

== system tadpole_dynamic_open_loop1/Vehicle Model/resistance calculation/Rear Traction add up/Fm<0/Switch Case Action Subsystem6/Switch Case Action Subsystem10 ==
  "value " : Inport
  Action Port : ActionPort  ActionPortLabel=case [ -1 ]:
  Gain : Gain  Gain=-1
  Out1 : Outport  VectorParamsAs1DForOutWhenUnconnected=off
  wires:
  Gain/1 -> Out1/1
  "value "/1 -> Gain/1

== system tadpole_dynamic_open_loop1/Vehicle Model/resistance calculation/Rear Traction add up/Fm<0/Switch Case Action Subsystem6/Switch Case Action Subsystem11 ==
  "value " : Inport
  Action Port : ActionPort  ActionPortLabel=default:
  Out1 : Outport  VectorParamsAs1DForOutWhenUnconnected=off
  wires:
  "value "/1 -> Out1/1

== system tadpole_dynamic_open_loop1/Vehicle Model/resistance calculation/Rear Traction add up/Fm<0/Switch Case Action Subsystem6/Switch Case Action Subsystem9 ==
  "value " : Inport
  Action Port : ActionPort  ActionPortLabel=case [ 1 ]:
  Gain : Gain  Gain=-1
  Out1 : Outport  VectorParamsAs1DForOutWhenUnconnected=off
  wires:
  "value "/1 -> Gain/1
  Gain/1 -> Out1/1

== system tadpole_dynamic_open_loop1/Vehicle Model/resistance calculation/Rear Traction add up/Fm<0/Switch Case Action Subsystem7/Switch Case Action Subsystem12 ==
  "value " : Inport
  Action Port : ActionPort  ActionPortLabel=case [ -1 ]:
  Out1 : Outport  VectorParamsAs1DForOutWhenUnconnected=off
  wires:
  "value "/1 -> Out1/1

== system tadpole_dynamic_open_loop1/Vehicle Model/resistance calculation/Rear Traction add up/Fm<0/Switch Case Action Subsystem7/Switch Case Action Subsystem13 ==
  "value " : Inport
  Action Port : ActionPort  ActionPortLabel=default:
  Out1 : Outport  VectorParamsAs1DForOutWhenUnconnected=off
  wires:
  "value "/1 -> Out1/1

== system tadpole_dynamic_open_loop1/Vehicle Model/resistance calculation/Rear Traction add up/Fm<0/Switch Case Action Subsystem7/Switch Case Action Subsystem14 ==
  "value " : Inport
  Action Port : ActionPort  ActionPortLabel=case [ 1 ]:
  Out1 : Outport  VectorParamsAs1DForOutWhenUnconnected=off
  wires:
  "value "/1 -> Out1/1

== system tadpole_dynamic_open_loop1/Vehicle Model/resistance calculation/Rear Traction add up/Fm>=0/Switch Case Action Subsystem6/Switch Case Action Subsystem10 ==
  "value " : Inport
  Action Port : ActionPort  ActionPortLabel=case [ -1 ]:
  Gain : Gain  Gain=-1
  Out1 : Outport  VectorParamsAs1DForOutWhenUnconnected=off
  wires:
  Gain/1 -> Out1/1
  "value "/1 -> Gain/1

== system tadpole_dynamic_open_loop1/Vehicle Model/resistance calculation/Rear Traction add up/Fm>=0/Switch Case Action Subsystem6/Switch Case Action Subsystem11 ==
  "value " : Inport
  Action Port : ActionPort  ActionPortLabel=default:
  Out1 : Outport  VectorParamsAs1DForOutWhenUnconnected=off
  wires:
  "value "/1 -> Out1/1

== system tadpole_dynamic_open_loop1/Vehicle Model/resistance calculation/Rear Traction add up/Fm>=0/Switch Case Action Subsystem6/Switch Case Action Subsystem9 ==
  "value " : Inport
  Action Port : ActionPort  ActionPortLabel=case [ 1 ]:
  Out1 : Outport  VectorParamsAs1DForOutWhenUnconnected=off
  wires:
  "value "/1 -> Out1/1

== system tadpole_dynamic_open_loop1/Vehicle Model/resistance calculation/Rear Traction add up/Fm>=0/Switch Case Action Subsystem7/Switch Case Action Subsystem12 ==
  "value " : Inport
  Action Port : ActionPort  ActionPortLabel=case [ -1 ]:
  Gain : Gain  Gain=-1
  Out1 : Outport  VectorParamsAs1DForOutWhenUnconnected=off
  wires:
  "value "/1 -> Gain/1
  Gain/1 -> Out1/1

== system tadpole_dynamic_open_loop1/Vehicle Model/resistance calculation/Rear Traction add up/Fm>=0/Switch Case Action Subsystem7/Switch Case Action Subsystem13 ==
  "value " : Inport
  Action Port : ActionPort  ActionPortLabel=default:
  Out1 : Outport  VectorParamsAs1DForOutWhenUnconnected=off
  wires:
  "value "/1 -> Out1/1

== system tadpole_dynamic_open_loop1/Vehicle Model/resistance calculation/Rear Traction add up/Fm>=0/Switch Case Action Subsystem7/Switch Case Action Subsystem14 ==
  "value " : Inport
  Action Port : ActionPort  ActionPortLabel=case [ 1 ]:
  Out1 : Outport  VectorParamsAs1DForOutWhenUnconnected=off
  wires:
  "value "/1 -> Out1/1

== system tadpole_dynamic_open_loop1/Vehicle Model/resistance calculation/Rear Traction add up/Fm>=0/m>b/Switch Case Action Subsystem6 ==
  "value " : Inport
  Action Port : ActionPort  ActionPortLabel=case [ 1 ]:
  Out1 : Outport  VectorParamsAs1DForOutWhenUnconnected=off
  wires:
  "value "/1 -> Out1/1

== system tadpole_dynamic_open_loop1/Vehicle Model/resistance calculation/Rear Traction add up/Fm>=0/m>b/Switch Case Action Subsystem7 ==
  "value " : Inport
  Action Port : ActionPort  ActionPortLabel=case [ -1 ]:
  Gain : Gain  Gain=-1
  Out1 : Outport  VectorParamsAs1DForOutWhenUnconnected=off
  wires:
  "value "/1 -> Gain/1
  Gain/1 -> Out1/1

== system tadpole_dynamic_open_loop1/Vehicle Model/resistance calculation/Rear Traction add up/Fm>=0/m>b/Switch Case Action Subsystem8 ==
  "value " : Inport
  Action Port : ActionPort  ActionPortLabel=default:
  Out1 : Outport  VectorParamsAs1DForOutWhenUnconnected=off
  wires:
  "value "/1 -> Out1/1

== system tadpole_dynamic_open_loop1/Vehicle Model/Tadpole vehicle dynamic/Calculation/Side slip angle Rear/velocity limit1/If Action Subsystem2/If Action Subsystem ==
  In1 : Inport
  Action Port : ActionPort  ActionPortLabel=if(0.0005>u1 )
  Out1 : Outport  VectorParamsAs1DForOutWhenUnconnected=off
  wires:
  In1/1 -> Out1/1

== system tadpole_dynamic_open_loop1/Vehicle Model/Tadpole vehicle dynamic/Calculation/Side slip angle Rear/velocity limit1/If Action Subsystem2/If Action Subsystem1 ==
  In1 : Inport
  Action Port : ActionPort  ActionPortLabel=else
  Out1 : Outport  VectorParamsAs1DForOutWhenUnconnected=off
  wires:
  In1/1 -> Out1/1

== system tadpole_dynamic_open_loop1/Vehicle Model/Tadpole vehicle dynamic/Calculation/Side slip angle Rear/velocity limit1/If Action Subsystem3/If Action Subsystem ==
  In1 : Inport
  Action Port : ActionPort  ActionPortLabel=if(-0.0005<u1 )
  Out1 : Outport  VectorParamsAs1DForOutWhenUnconnected=off
  wires:
  In1/1 -> Out1/1

== system tadpole_dynamic_open_loop1/Vehicle Model/Tadpole vehicle dynamic/Calculation/Side slip angle Rear/velocity limit1/If Action Subsystem3/If Action Subsystem1 ==
  In1 : Inport
  Action Port : ActionPort  ActionPortLabel=else
  Out1 : Outport  VectorParamsAs1DForOutWhenUnconnected=off
  wires:
  In1/1 -> Out1/1

== system tadpole_dynamic_open_loop1/Vehicle Model/Tadpole vehicle dynamic/Calculation/Subsystem1/Subsystem/linear slip cal fR /slip recgonition ==
  In2 : Inport
  In3 : Inport  Port=2
  Constant : Constant
  Constant1 : Constant  Value=-1
  If : If  IfExpression=u1~=0
  If Action Subsystem : Subsystem  TreatAsAtomicUnit=on
  If Action Subsystem1 : Subsystem  TreatAsAtomicUnit=on
  Merge : Merge
  Subtract : Sum  Inputs=+-
  tag scope: Force_lateral_slip_reg_fR=global
  wires:
  Constant/1 -> If Action Subsystem/1(In1)
  If/1 -> If Action Subsystem/Action
  Subtract/1 -> If/1
  If Action Subsystem/1(Out1) -> Merge/1
  In2/1 -> Subtract/1
  If/2 -> If Action Subsystem1/Action
  In3/1 -> Subtract/2
  If Action Subsystem1/1(Out1) -> Merge/2
  Constant1/1 -> If Action Subsystem1/1(In1)
  Merge/1 -> [Force_lateral_slip_reg_fR]

== system tadpole_dynamic_open_loop1/Vehicle Model/Tadpole vehicle dynamic/Calculation/Subsystem1/velocity limit/If Action Subsystem2/If Action Subsystem ==
  In1 : Inport
  Action Port : ActionPort
  Out1 : Outport  VectorParamsAs1DForOutWhenUnconnected=off
  wires:
  In1/1 -> Out1/1

== system tadpole_dynamic_open_loop1/Vehicle Model/Tadpole vehicle dynamic/Calculation/Subsystem1/velocity limit/If Action Subsystem2/If Action Subsystem1 ==
  In1 : Inport
  Action Port : ActionPort
  Out1 : Outport  VectorParamsAs1DForOutWhenUnconnected=off
  wires:
  In1/1 -> Out1/1

== system tadpole_dynamic_open_loop1/Vehicle Model/Tadpole vehicle dynamic/Calculation/Subsystem1/velocity limit/If Action Subsystem3/If Action Subsystem ==
  In1 : Inport
  Action Port : ActionPort
  Out1 : Outport  VectorParamsAs1DForOutWhenUnconnected=off
  wires:
  In1/1 -> Out1/1

== system tadpole_dynamic_open_loop1/Vehicle Model/Tadpole vehicle dynamic/Calculation/Subsystem1/velocity limit/If Action Subsystem3/If Action Subsystem1 ==
  In1 : Inport
  Action Port : ActionPort
  Out1 : Outport  VectorParamsAs1DForOutWhenUnconnected=off
  wires:
  In1/1 -> Out1/1

== system tadpole_dynamic_open_loop1/Vehicle Model/Tadpole vehicle dynamic/Calculation/Subsystem2/Subsystem/linear slip cal r /slip recgonition ==
  In2 : Inport
  In3 : Inport  Port=2
  Constant : Constant
  Constant1 : Constant  Value=-1
  If : If  IfExpression=u1~=0
  If Action Subsystem : Subsystem  TreatAsAtomicUnit=on
  If Action Subsystem1 : Subsystem  TreatAsAtomicUnit=on
  Merge : Merge
  Subtract : Sum  Inputs=+-
  tag scope: Force_lateral_slip_reg_r=global
  wires:
  Constant/1 -> If Action Subsystem/1(In1)
  If/1 -> If Action Subsystem/Action
  Subtract/1 -> If/1
  If Action Subsystem/1(Out1) -> Merge/1
  In2/1 -> Subtract/1
  If/2 -> If Action Subsystem1/Action
  In3/1 -> Subtract/2
  If Action Subsystem1/1(Out1) -> Merge/2
  Constant1/1 -> If Action Subsystem1/1(In1)
  Merge/1 -> [Force_lateral_slip_reg_r]

== system tadpole_dynamic_open_loop1/Vehicle Model/Tadpole vehicle dynamic/Calculation/Subsystem2/velocity limit/If Action Subsystem2/If Action Subsystem ==
  In1 : Inport
  Action Port : ActionPort
  Out1 : Outport  VectorParamsAs1DForOutWhenUnconnected=off
  wires:
  In1/1 -> Out1/1

== system tadpole_dynamic_open_loop1/Vehicle Model/Tadpole vehicle dynamic/Calculation/Subsystem2/velocity limit/If Action Subsystem2/If Action Subsystem1 ==
  In1 : Inport
  Action Port : ActionPort
  Out1 : Outport  VectorParamsAs1DForOutWhenUnconnected=off
  wires:
  In1/1 -> Out1/1

== system tadpole_dynamic_open_loop1/Vehicle Model/Tadpole vehicle dynamic/Calculation/Subsystem2/velocity limit/If Action Subsystem3/If Action Subsystem ==
  In1 : Inport
  Action Port : ActionPort
  Out1 : Outport  VectorParamsAs1DForOutWhenUnconnected=off
  wires:
  In1/1 -> Out1/1

== system tadpole_dynamic_open_loop1/Vehicle Model/Tadpole vehicle dynamic/Calculation/Subsystem2/velocity limit/If Action Subsystem3/If Action Subsystem1 ==
  In1 : Inport
  Action Port : ActionPort
  Out1 : Outport  VectorParamsAs1DForOutWhenUnconnected=off
  wires:
  In1/1 -> Out1/1

== system tadpole_dynamic_open_loop1/Vehicle Model/Tadpole vehicle dynamic/Calculation/Subsystem3/Subsystem/linear slip cal fL /slip recgonition ==
  In2 : Inport
  In3 : Inport  Port=2
  Constant : Constant
  Constant1 : Constant  Value=-1
  If : If  IfExpression=u1~=0
  If Action Subsystem : Subsystem  TreatAsAtomicUnit=on
  If Action Subsystem1 : Subsystem  TreatAsAtomicUnit=on
  Merge : Merge
  Subtract : Sum  Inputs=+-
  tag scope: Force_lateral_slip_reg_fL=global
  wires:
  Constant/1 -> If Action Subsystem/1(In1)
  If/1 -> If Action Subsystem/Action
  Subtract/1 -> If/1
  If Action Subsystem/1(Out1) -> Merge/1
  In2/1 -> Subtract/1
  If/2 -> If Action Subsystem1/Action
  In3/1 -> Subtract/2
  If Action Subsystem1/1(Out1) -> Merge/2
  Constant1/1 -> If Action Subsystem1/1(In1)
  Merge/1 -> [Force_lateral_slip_reg_fL]

== system tadpole_dynamic_open_loop1/Vehicle Model/Tadpole vehicle dynamic/Calculation/Subsystem3/velocity limit/If Action Subsystem2/If Action Subsystem ==
  In1 : Inport
  Action Port : ActionPort
  Out1 : Outport  VectorParamsAs1DForOutWhenUnconnected=off
  wires:
  In1/1 -> Out1/1

== system tadpole_dynamic_open_loop1/Vehicle Model/Tadpole vehicle dynamic/Calculation/Subsystem3/velocity limit/If Action Subsystem2/If Action Subsystem1 ==
  In1 : Inport
  Action Port : ActionPort
  Out1 : Outport  VectorParamsAs1DForOutWhenUnconnected=off
  wires:
  In1/1 -> Out1/1

== system tadpole_dynamic_open_loop1/Vehicle Model/Tadpole vehicle dynamic/Calculation/Subsystem3/velocity limit/If Action Subsystem3/If Action Subsystem ==
  In1 : Inport
  Action Port : ActionPort
  Out1 : Outport  VectorParamsAs1DForOutWhenUnconnected=off
  wires:
  In1/1 -> Out1/1

== system tadpole_dynamic_open_loop1/Vehicle Model/Tadpole vehicle dynamic/Calculation/Subsystem3/velocity limit/If Action Subsystem3/If Action Subsystem1 ==
  In1 : Inport
  Action Port : ActionPort
  Out1 : Outport  VectorParamsAs1DForOutWhenUnconnected=off
  wires:
  In1/1 -> Out1/1

== system tadpole_dynamic_open_loop1/Vehicle Model/Tadpole vehicle dynamic/Calculation/Subsystem4/Subsystem/linear slip cal fR /slip recgonition ==
  In2 : Inport
  In3 : Inport  Port=2
  Constant : Constant
  Constant1 : Constant  Value=-1
  If : If  IfExpression=u1~=0
  If Action Subsystem : Subsystem  TreatAsAtomicUnit=on
  If Action Subsystem1 : Subsystem  TreatAsAtomicUnit=on
  Merge : Merge
  Subtract : Sum  Inputs=+-
  tag scope: Force_lateral_slip_reg_fR=global
  wires:
  Constant/1 -> If Action Subsystem/1(In1)
  If/1 -> If Action Subsystem/Action
  Subtract/1 -> If/1
  If Action Subsystem/1(Out1) -> Merge/1
  In2/1 -> Subtract/1
  If/2 -> If Action Subsystem1/Action
  In3/1 -> Subtract/2
  If Action Subsystem1/1(Out1) -> Merge/2
  Constant1/1 -> If Action Subsystem1/1(In1)
  Merge/1 -> [Force_lateral_slip_reg_fR]

== system tadpole_dynamic_open_loop1/Vehicle Model/Tadpole vehicle dynamic/Calculation/Subsystem4/velocity limit/If Action Subsystem2/If Action Subsystem ==
  In1 : Inport
  Action Port : ActionPort  ActionPortLabel=if(0.005>u1 )
  Out1 : Outport  VectorParamsAs1DForOutWhenUnconnected=off
  wires:
  In1/1 -> Out1/1

== system tadpole_dynamic_open_loop1/Vehicle Model/Tadpole vehicle dynamic/Calculation/Subsystem4/velocity limit/If Action Subsystem2/If Action Subsystem1 ==
  In1 : Inport
  Action Port : ActionPort  ActionPortLabel=else
  Out1 : Outport  VectorParamsAs1DForOutWhenUnconnected=off
  wires:
  In1/1 -> Out1/1

== system tadpole_dynamic_open_loop1/Vehicle Model/Tadpole vehicle dynamic/Calculation/Subsystem4/velocity limit/If Action Subsystem3/If Action Subsystem ==
  In1 : Inport
  Action Port : ActionPort  ActionPortLabel=if(-0.005<u1 )
  Out1 : Outport  VectorParamsAs1DForOutWhenUnconnected=off
  wires:
  In1/1 -> Out1/1

== system tadpole_dynamic_open_loop1/Vehicle Model/Tadpole vehicle dynamic/Calculation/Subsystem4/velocity limit/If Action Subsystem3/If Action Subsystem1 ==
  In1 : Inport
  Action Port : ActionPort  ActionPortLabel=else
  Out1 : Outport  VectorParamsAs1DForOutWhenUnconnected=off
  wires:
  In1/1 -> Out1/1

== system tadpole_dynamic_open_loop1/Vehicle Model/Tadpole vehicle dynamic/Calculation/Subsystem5/Subsystem/linear slip cal r /slip recgonition ==
  In2 : Inport
  In3 : Inport  Port=2
  Constant : Constant
  Constant1 : Constant  Value=-1
  If : If  IfExpression=u1~=0
  If Action Subsystem : Subsystem  TreatAsAtomicUnit=on
  If Action Subsystem1 : Subsystem  TreatAsAtomicUnit=on
  Merge : Merge
  Subtract : Sum  Inputs=+-
  tag scope: Force_lateral_slip_reg_r=global
  wires:
  Constant/1 -> If Action Subsystem/1(In1)
  If/1 -> If Action Subsystem/Action
  Subtract/1 -> If/1
  If Action Subsystem/1(Out1) -> Merge/1
  In2/1 -> Subtract/1
  If/2 -> If Action Subsystem1/Action
  In3/1 -> Subtract/2
  If Action Subsystem1/1(Out1) -> Merge/2
  Constant1/1 -> If Action Subsystem1/1(In1)
  Merge/1 -> [Force_lateral_slip_reg_r]

== system tadpole_dynamic_open_loop1/Vehicle Model/Tadpole vehicle dynamic/Calculation/Subsystem5/velocity limit/If Action Subsystem2/If Action Subsystem ==
  In1 : Inport
  Action Port : ActionPort  ActionPortLabel=if(0.005>u1 )
  Out1 : Outport  VectorParamsAs1DForOutWhenUnconnected=off
  wires:
  In1/1 -> Out1/1

== system tadpole_dynamic_open_loop1/Vehicle Model/Tadpole vehicle dynamic/Calculation/Subsystem5/velocity limit/If Action Subsystem2/If Action Subsystem1 ==
  In1 : Inport
  Action Port : ActionPort  ActionPortLabel=else
  Out1 : Outport  VectorParamsAs1DForOutWhenUnconnected=off
  wires:
  In1/1 -> Out1/1

== system tadpole_dynamic_open_loop1/Vehicle Model/Tadpole vehicle dynamic/Calculation/Subsystem5/velocity limit/If Action Subsystem3/If Action Subsystem ==
  In1 : Inport
  Action Port : ActionPort  ActionPortLabel=if(-0.005<u1 )
  Out1 : Outport  VectorParamsAs1DForOutWhenUnconnected=off
  wires:
  In1/1 -> Out1/1
